simulink model "fwv_fulatti"  (R2021b)
settings: Solver=ode15s  StartTime=0.0  StopTime=10  FixedStep=0.01  MaxStep=0.01  RelTol=1e-3  AbsTol=1e-3  EnableMultiTasking=on
model workspace (MATLAB code in the model file):
  | p0=[0 0 0];
values from neighbouring files (symbols this model uses):
  A_D = 1.5    [main.m]    (also in param.m; params.m)
  A_L = 1.8    [main.m]    (also in param.m; params.m)
  c_bar = S/R    (= 0.0357142857143)    [main.m]    (also in param.m = 0.0251327412287; params.m)
  C_D0 = 0.45    [main.m]    (also in param.m; params.m)
  m = 2    [rbf_pid.m]
  r00 = double(int(f,[0,1]))    [main.m]    (also in param.m = 1; params.m = 0.933333333333)
  r11 = double(int(x*f,[0,1]))    [main.m]    (also in param.m = double(int(curv(x)*(x+1/9),0,1)); params.m = 0.481185185185)
  r22 = double(int(x^2*f,[0,1]))    [main.m]    (also in param.m = double(int(curv(x)*(x+1/9)^2,0,1)); params.m = 0.304750617284)
  r33 = double(int(x^3*f,[0,1]))    [main.m]    (also in param.m = double(int(curv(x)*(x+1/9)^3,0,1)); params.m = 0.218568691358)
  r_cp = Rw*r33/r22    [main.m]    (also in param.m; params.m = 0.10758076225)
  rho = 1.205    [main.m]    (also in param.m; params.m)
  Rw = 0.15    [main.m]    (also in param.m = 0.075; params.m)
  z00 = double(int(f^2,[0,1]))    [main.m]    (also in param.m = double(int(curv(x)^2,0,1)); params.m = 1.00177777778)
  z11 = double(int(x*f^2,[0,1]))    [main.m]    (also in param.m = double(int(curv(x)^2*(x+1/9),0,1)); params.m = 0.484918518519)
  z22 = double(int(x^2*f^2,[0,1]))    [main.m]    (also in param.m = double(int(curv(x)^2*(x+1/9)^2,0,1)); params.m = 0.28785382716)
  zrd = double(int(f^4,[0,1]))    [main.m]    (also in param.m = double(int(curv(x)^4,0,1)); params.m = 1.29333866667)
undefined symbols (not defined in the file or in its folder): X, Y, Z
libraries: sm_lib x57, nesl_utility x45, vrlib x3, slpidlib x2
(part 3 of 3)

== system fwv_fulatti/Controller/Outer PD ==
  ep : Inport
  ev : Inport  Port=2
  a : Inport  Port=3
  Demux : Demux  Outputs=3
  Demux1 : Demux  Outputs=3
  Demux2 : Demux  Outputs=3
  x PD : Subsystem  mask{Kp=6, Ki=0, Kd=3}
  x PID : slpidlib/PID Controller  Commented=on  Controller=PID  Form=Parallel  TimeDomain=Continuous-time  UseExternalTs=off  SampleTime=-1  IntegratorMethod=Forward Euler  FilterMethod=Forward Euler  ControllerParametersSource=internal  P=0.5  I=0  D=0.1  UseFilter=on  N=25  TunerSelectOption=Transfer Function Based (PID Tuner App)  InitialConditionSource=internal  InitialConditionForIntegrator=0  InitialConditionForFilter=0  DifferentiatorICPrevScaledInput=0  ExternalReset=none  TrackingMode=off  Kt=1  LimitOutput=off  SatLimitsSource=internal  UpperSaturationLimit=0.5  LowerSaturationLimit=-0.5  LinearizeAsGain=on  AntiWindupMode=none  Kb=1  POutMin=[]  POutMax=[]  IOutMin=[]  IOutMax=[]  DOutMin=[]  DOutMax=[]  NOutMin=[]  NOutMax=[]  SumOutDataTypeStr=double  SumOutMin=[]  SumOutMax=[]  SaturationOutMin=[]  SaturationOutMax=[]  PParamMin=[]  PParamMax=[]  IParamMin=[]  IParamMax=[]  DParamMin=[]  DParamMax=[]  NParamMin=[]  NParamMax=[]  KbParamMin=[]  KbParamMax=[]  KtParamMin=[]  KtParamMax=[]  KbOutMin=[]  KbOutMax=[]  KtOutMin=[]  KtOutMax=[]  IntegratorOutMin=[]  IntegratorOutMax=[]  FilterOutMin=[]  FilterOutMax=[]  SumI1OutMin=[]  SumI1OutMax=[]  SumI2OutMin=[]  SumI2OutMax=[]  SumI3OutMin=[]  SumI3OutMax=[]  SumI4OutMin=[]  SumI4OutMax=[]  SumDOutMin=[]  SumDOutMax=[]  DifferentiatorOutMin=[]  DifferentiatorOutMax=[]  FilterDiffOutCoefMin=[]  FilterDiffOutCoefMax=[]  ReciprocalOutMin=[]  ReciprocalOutMax=[]  SumDenOutMin=[]  SumDenOutMax=[]  SumNumOutMin=[]  SumNumOutMax=[]  DivideOutMin=[]  DivideOutMax=[]  UdiffTsProdOutMin=[]  UdiffTsProdOutMax=[]  NTsProdOutMin=[]  NTsProdOutMax=[]  UintegralTsProdOutMin=[]  UintegralTsProdOutMax=[]  UngainTsProdOutMin=[]  UngainTsProdOutMax=[]  IntegratorContinuousStateAttributes=''  IntegratorStateMustResolveToSignalObject=off  IntegratorRTWStateStorageClass=Auto  FilterContinuousStateAttributes=''  FilterStateMustResolveToSignalObject=off  FilterRTWStateStorageClass=Auto  ParallelPVariant=InternalParameters  IdealPVariant=Disabled  IVariant=InternalParameters  DVariant=InternalParameters  IntegratorVariant=Continuous  SatVariant=Disabled  AWVariant=Passthrough  PCopyVariant=Disabled  TRVariant=Disabled  FdbkBlocksVariant=Forward  IdealPFdbkVariant=Disabled  SatFdbkVariant=Disabled  DerivativeFilterVariant=ContFilter  NVariant=InternalParameters  NCopyVariant=Disabled  FilterICVariant=InternalICsFilter  IntegratorICVariant=InternalICs  ExternalResetVariant=Disabled  TRSumVariant=Passthrough  SumFdbkVariant=Disabled  SumVariant=Sum_PID  TsampFilterVariant=InternalTs  TsampNgainVariant=Passthrough  TsampIntegralVariant=Passthrough  ExternalSaturationOutDataTypeStr=Inherit: Same as second input
  y PD : Subsystem  mask{Kp=6, Ki=0, Kd=6}
  y PID : slpidlib/PID Controller  Commented=on  Controller=PID  Form=Parallel  TimeDomain=Continuous-time  UseExternalTs=off  SampleTime=-1  IntegratorMethod=Forward Euler  FilterMethod=Forward Euler  ControllerParametersSource=internal  P=0.3  I=0  D=0.3  UseFilter=on  N=25  TunerSelectOption=Transfer Function Based (PID Tuner App)  InitialConditionSource=internal  InitialConditionForIntegrator=0  InitialConditionForFilter=0  DifferentiatorICPrevScaledInput=0  ExternalReset=none  TrackingMode=off  Kt=1  LimitOutput=off  SatLimitsSource=internal  UpperSaturationLimit=0.5  LowerSaturationLimit=-0.5  LinearizeAsGain=on  AntiWindupMode=none  Kb=1  POutMin=[]  POutMax=[]  IOutMin=[]  IOutMax=[]  DOutMin=[]  DOutMax=[]  NOutMin=[]  NOutMax=[]  SumOutMin=[]  SumOutMax=[]  SaturationOutMin=[]  SaturationOutMax=[]  PParamMin=[]  PParamMax=[]  IParamMin=[]  IParamMax=[]  DParamMin=[]  DParamMax=[]  NParamMin=[]  NParamMax=[]  KbParamMin=[]  KbParamMax=[]  KtParamMin=[]  KtParamMax=[]  KbOutMin=[]  KbOutMax=[]  KtOutMin=[]  KtOutMax=[]  IntegratorOutMin=[]  IntegratorOutMax=[]  FilterOutMin=[]  FilterOutMax=[]  SumI1OutMin=[]  SumI1OutMax=[]  SumI2OutMin=[]  SumI2OutMax=[]  SumI3OutMin=[]  SumI3OutMax=[]  SumI4OutMin=[]  SumI4OutMax=[]  SumDOutMin=[]  SumDOutMax=[]  DifferentiatorOutMin=[]  DifferentiatorOutMax=[]  FilterDiffOutCoefMin=[]  FilterDiffOutCoefMax=[]  ReciprocalOutMin=[]  ReciprocalOutMax=[]  SumDenOutMin=[]  SumDenOutMax=[]  SumNumOutMin=[]  SumNumOutMax=[]  DivideOutMin=[]  DivideOutMax=[]  UdiffTsProdOutMin=[]  UdiffTsProdOutMax=[]  NTsProdOutMin=[]  NTsProdOutMax=[]  UintegralTsProdOutMin=[]  UintegralTsProdOutMax=[]  UngainTsProdOutMin=[]  UngainTsProdOutMax=[]  IntegratorContinuousStateAttributes=''  IntegratorStateMustResolveToSignalObject=off  IntegratorRTWStateStorageClass=Auto  FilterContinuousStateAttributes=''  FilterStateMustResolveToSignalObject=off  FilterRTWStateStorageClass=Auto  ParallelPVariant=InternalParameters  IdealPVariant=Disabled  IVariant=InternalParameters  DVariant=InternalParameters  IntegratorVariant=Continuous  SatVariant=Disabled  AWVariant=Passthrough  PCopyVariant=Disabled  TRVariant=Disabled  FdbkBlocksVariant=Forward  IdealPFdbkVariant=Disabled  SatFdbkVariant=Disabled  DerivativeFilterVariant=ContFilter  NVariant=InternalParameters  NCopyVariant=Disabled  FilterICVariant=InternalICsFilter  IntegratorICVariant=InternalICs  ExternalResetVariant=Disabled  TRSumVariant=Passthrough  SumFdbkVariant=Disabled  SumVariant=Sum_PID  TsampFilterVariant=InternalTs  TsampNgainVariant=Passthrough  TsampIntegralVariant=Passthrough  ExternalSaturationOutDataTypeStr=Inherit: Same as second input
  z PD : Subsystem  mask{Kp=10, Ki=0, Kd=4}
  mux : Outport
  muy : Outport  Port=2
  muz : Outport  Port=3
  wires:
  ep/1 -> Demux/1
  ev/1 -> Demux1/1
  x PD/1(Out1) -> mux/1
  y PD/1(Out1) -> muy/1
  z PD/1(Out1) -> muz/1
  a/1 -> Demux2/1
  Demux1/2 -> y PD/2(In2)
  Demux2/3 -> z PD/3(In3)
  Demux2/2 -> y PD/3(In3)
  Demux1/1 -> x PD/2(In2)
  Demux1/3 -> z PD/2(In2)
  Demux/3 -> z PD/1(In1)
  Demux2/1 -> x PD/3(In3)
  Demux/1 -> x PD/1(In1)
  Demux/2 -> y PD/1(In1)

== system fwv_fulatti/Controller/R to euler ==
  R : Inport
  Mux : Mux  Inputs=3
  R to X-Y-Z Extrinsic : Subsystem  mask(Rotation Matrix to X-Y-Z Extrinsic){}
      mask help: Computes roll / pitch / yaw values assuming they correspond to X, Y, and Z rotations, applied in that order and using extrinsic rotations (rotations applied about the fixed axes of the base frame). Does not handle case where Y (pitch) rotation is +/-90 degrees.
  Terminator : Terminator
  rad2deg : Gain  Gain=180/pi
  wires:
  R/1 -> R to X-Y-Z Extrinsic/1(R)
  R to X-Y-Z Extrinsic/2(pitch) -> Mux/2
  Mux/1 -> rad2deg/1
  rad2deg/1 -> Terminator/1
  R to X-Y-Z Extrinsic/1(roll) -> Mux/1
  R to X-Y-Z Extrinsic/3(yaw) -> Mux/3

== system fwv_fulatti/Controller/Rd to euler ==
  R : Inport
  Mux : Mux  Inputs=3
  R to X-Y-Z Extrinsic : Subsystem  mask(Rotation Matrix to X-Y-Z Extrinsic){}
      mask help: Computes roll / pitch / yaw values assuming they correspond to X, Y, and Z rotations, applied in that order and using extrinsic rotations (rotations applied about the fixed axes of the base frame). Does not handle case where Y (pitch) rotation is +/-90 degrees.
  Terminator : Terminator
  rad2deg : Gain  Gain=180/pi
  wires:
  rad2deg/1 -> Terminator/1
  R/1 -> R to X-Y-Z Extrinsic/1(R)
  Mux/1 -> rad2deg/1
  R to X-Y-Z Extrinsic/3(yaw) -> Mux/3
  R to X-Y-Z Extrinsic/1(roll) -> Mux/1
  R to X-Y-Z Extrinsic/2(pitch) -> Mux/2

== system fwv_fulatti/Controller/adaptive mapping estimator ==
  mu : Inport
  Integrator : Integrator  InitialCondition=0.05
  update k_hat : MATLAB Function  TreatAsAtomicUnit=on
  k_hat : Outport
  wires:
  update k_hat/1(k_hat_dot) -> Integrator/1
  mu/1 -> update k_hat/1(mu)
  Integrator/1 -> update k_hat/2(k_hat), k_hat/1

== system fwv_fulatti/Controller/averaged R to euler ==
  R : Inport
  Mux : Mux  Inputs=3
  R to X-Y-Z Extrinsic : Subsystem  mask(Rotation Matrix to X-Y-Z Extrinsic){}
      mask help: Computes roll / pitch / yaw values assuming they correspond to X, Y, and Z rotations, applied in that order and using extrinsic rotations (rotations applied about the fixed axes of the base frame). Does not handle case where Y (pitch) rotation is +/-90 degrees.
  Terminator : Terminator
  rad2deg : Gain  Gain=180/pi
  wires:
  R/1 -> R to X-Y-Z Extrinsic/1(R)
  R to X-Y-Z Extrinsic/2(pitch) -> Mux/2
  Mux/1 -> rad2deg/1
  rad2deg/1 -> Terminator/1
  R to X-Y-Z Extrinsic/1(roll) -> Mux/1
  R to X-Y-Z Extrinsic/3(yaw) -> Mux/3

== system fwv_fulatti/Controller/period averaging ==
  in : Inport
  MATLAB Function : MATLAB Function  TreatAsAtomicUnit=on
  Mean : Subsystem
  Mean1 : Outport
  wires:
  in/1 -> Mean/1(In1)
  Mean/1(Out1) -> MATLAB Function/1(R_raw)
  MATLAB Function/1(R_mean) -> Mean1/1

== system fwv_fulatti/Body/LEFT WING/Subsystem1 ==
  Gain : Gain  Gain=-1
  LWing-root in world : sm_lib/Frames and Transforms/Transform Sensor  MeasurementFrame=NonRotatingFollower  SenseAngle=off  SenseAxis=off  SenseAngle1=off  SenseAngle2=off  SenseAngle3=off  SenseQ=off  SenseR=off  SenseOmegaX=on  SenseOmegaY=on  SenseOmegaZ=off  SenseOmega1=off  SenseOmega2=off  SenseOmega3=off  SenseQDot=off  SenseRDot=off  SenseAlphaX=off  SenseAlphaY=off  SenseAlphaZ=off  SenseAlpha1=off  SenseAlpha2=off  SenseAlpha3=off  SenseQDDot=off  SenseRDDot=off  SenseX=off  SenseY=off  SenseZ=off  SenseRad=off  SenseAzim=off  SenseDist=off  SenseInc=off  SenseXDot=on  SenseYDot=on  SenseZDot=off  SenseRadDot=off  SenseAzimDot=off  SenseDistDot=off  SenseIncDot=off  SenseXDDot=off  SenseYDDot=off  SenseZDDot=off  SenseRadDDot=off  SenseAzimDDot=off  SenseDistDDot=off  SenseIncDDot=off
  Mux : Mux
  PS-Simulink Converter{,1..3} (4 alike) : nesl_utility/PS-Simulink Converter  PhysicalDomain=network_engine_domain  SubClassName=ps_output  LeftPortType=input  RightPortType=output  PseudoPeriodic=off  Frequencies=[]  Unit=inherit  AffineConversion=off
      settings: SourceProductBaseCode=PW,SS
  W : PMIOPort  Side=Left
  WT : PMIOPort  Port=2  Side=Left
  le0 : Outport
  wires:
  Mux/1 -> le0/1
  Gain/1 -> Mux/2
  PS-Simulink Converter1/1 -> Mux/3
  PS-Simulink Converter3/1 -> Gain/1
  PS-Simulink Converter2/1 -> Mux/1
  PS-Simulink Converter/1 -> Mux/4
  connections:
  W/RConn1 -- LWing-root in world/LConn1
  WT/RConn1 -- LWing-root in world/RConn1
  LWing-root in world/RConn2 -- PS-Simulink Converter/LConn1
  LWing-root in world/RConn3 -- PS-Simulink Converter1/LConn1
  LWing-root in world/RConn4 -- PS-Simulink Converter2/LConn1
  LWing-root in world/RConn5 -- PS-Simulink Converter3/LConn1

== system fwv_fulatti/Body/RIGHT WING/Subsystem1 ==
  Gain : Gain  Gain=-1
  LWing-root in world : sm_lib/Frames and Transforms/Transform Sensor  MeasurementFrame=NonRotatingFollower  SenseAngle=off  SenseAxis=off  SenseAngle1=off  SenseAngle2=off  SenseAngle3=off  SenseQ=off  SenseR=off  SenseOmegaX=on  SenseOmegaY=on  SenseOmegaZ=off  SenseOmega1=off  SenseOmega2=off  SenseOmega3=off  SenseQDot=off  SenseRDot=off  SenseAlphaX=off  SenseAlphaY=off  SenseAlphaZ=off  SenseAlpha1=off  SenseAlpha2=off  SenseAlpha3=off  SenseQDDot=off  SenseRDDot=off  SenseX=off  SenseY=off  SenseZ=off  SenseRad=off  SenseAzim=off  SenseDist=off  SenseInc=off  SenseXDot=on  SenseYDot=on  SenseZDot=off  SenseRadDot=off  SenseAzimDot=off  SenseDistDot=off  SenseIncDot=off  SenseXDDot=off  SenseYDDot=off  SenseZDDot=off  SenseRadDDot=off  SenseAzimDDot=off  SenseDistDDot=off  SenseIncDDot=off
  Mux : Mux
  PS-Simulink Converter{,1..3} (4 alike) : nesl_utility/PS-Simulink Converter  PhysicalDomain=network_engine_domain  SubClassName=ps_output  LeftPortType=input  RightPortType=output  PseudoPeriodic=off  Frequencies=[]  Unit=inherit  AffineConversion=off
      settings: SourceProductBaseCode=PW,SS
  W : PMIOPort  Side=Left
  WT : PMIOPort  Port=2  Side=Left
  le0 : Outport
  wires:
  Mux/1 -> le0/1
  Gain/1 -> Mux/2
  PS-Simulink Converter1/1 -> Mux/3
  PS-Simulink Converter3/1 -> Gain/1
  PS-Simulink Converter2/1 -> Mux/1
  PS-Simulink Converter/1 -> Mux/4
  connections:
  W/RConn1 -- LWing-root in world/LConn1
  WT/RConn1 -- LWing-root in world/RConn1
  LWing-root in world/RConn2 -- PS-Simulink Converter/LConn1
  LWing-root in world/RConn3 -- PS-Simulink Converter1/LConn1
  LWing-root in world/RConn4 -- PS-Simulink Converter2/LConn1
  LWing-root in world/RConn5 -- PS-Simulink Converter3/LConn1

== system fwv_fulatti/Controller/Inner PD/get P ==
  eR : Inport
  Add : Sum  Inputs=+++
  Cross Product : vrlib/Utilities/Cross Product
  Cross Product1 : vrlib/Utilities/Cross Product
  Cross Product2 : vrlib/Utilities/Cross Product
  One : Constant  Value=[1;0;0]  OutDataTypeStr=Inherit: Inherit via back propagation
  One1 : Constant  Value=[0;1;0]  OutDataTypeStr=Inherit: Inherit via back propagation
  One2 : Constant  Value=[0;0;1]  OutDataTypeStr=Inherit: Inherit via back propagation
  Product : Product  Multiplication=Matrix(*)
  Product1 : Product  Multiplication=Matrix(*)
  Product2 : Product  Multiplication=Matrix(*)
  Out : Outport
  wires:
  One/1 -> Product/2, Cross Product/1
  One1/1 -> Cross Product1/1, Product1/2
  One2/1 -> Cross Product2/1, Product2/2
  eR/1 -> Product/1, Product1/1, Product2/1
  Cross Product/1 -> Add/1
  Cross Product1/1 -> Add/2
  Cross Product2/1 -> Add/3
  Add/1 -> Out/1
  Product/1 -> Cross Product/2
  Product1/1 -> Cross Product1/2
  Product2/1 -> Cross Product2/2

== system fwv_fulatti/Controller/Inner PD/to euler1 ==
  R : Inport
  Mux : Mux  Inputs=3
  R to X-Y-Z Extrinsic : Subsystem  mask(Rotation Matrix to X-Y-Z Extrinsic){}
      mask help: Computes roll / pitch / yaw values assuming they correspond to X, Y, and Z rotations, applied in that order and using extrinsic rotations (rotations applied about the fixed axes of the base frame). Does not handle case where Y (pitch) rotation is +/-90 degrees.
  Terminator : Terminator
  rad2deg : Gain  Gain=180/pi
  wires:
  rad2deg/1 -> Terminator/1
  R/1 -> R to X-Y-Z Extrinsic/1(R)
  Mux/1 -> rad2deg/1
  R to X-Y-Z Extrinsic/3(yaw) -> Mux/3
  R to X-Y-Z Extrinsic/1(roll) -> Mux/1
  R to X-Y-Z Extrinsic/2(pitch) -> Mux/2

== system fwv_fulatti/Controller/Outer PD/x PD ==
  In1 : Inport
  In2 : Inport  Port=2
  In3 : Inport  Port=3
  Add : Sum  Inputs=++++
  Constant : Constant  Value=Kp
  Constant1 : Constant  Value=Ki
  Constant2 : Constant  Value=Kd
  Gain : Gain
  Integrator Limited : Integrator  UpperSaturationLimit=1  LowerSaturationLimit=0
  Product : Product
  Product1 : Product
  Product2 : Product
  Scope : Scope  NumInputPorts=2
  Out1 : Outport
  wires:
  Add/1 -> Out1/1
  In1/1 -> Product1/2, Product/2
  Product/1 -> Scope/1, Add/1
  Constant/1 -> Product/1
  Product2/1 -> Scope/2, Add/3
  In2/1 -> Product2/2
  Constant2/1 -> Product2/1
  Integrator Limited/1 -> Add/2
  Product1/1 -> Integrator Limited/1
  Constant1/1 -> Product1/1
  In3/1 -> Gain/1
  Gain/1 -> Add/4

== system fwv_fulatti/Controller/Outer PD/y PD ==
  In1 : Inport
  In2 : Inport  Port=2
  In3 : Inport  Port=3
  Add : Sum  Inputs=++++
  Constant : Constant  Value=Kp
  Constant1 : Constant  Value=Ki
  Constant2 : Constant  Value=Kd
  Gain : Gain
  Integrator Limited : Integrator  UpperSaturationLimit=1  LowerSaturationLimit=0
  Product : Product
  Product1 : Product
  Product2 : Product
  Out1 : Outport
  wires:
  Add/1 -> Out1/1
  In1/1 -> Product1/2, Product/2
  Product/1 -> Add/1
  Constant/1 -> Product/1
  Product2/1 -> Add/3
  In2/1 -> Product2/2
  Constant2/1 -> Product2/1
  Integrator Limited/1 -> Add/2
  Product1/1 -> Integrator Limited/1
  Constant1/1 -> Product1/1
  In3/1 -> Gain/1
  Gain/1 -> Add/4

== system fwv_fulatti/Controller/Outer PD/z PD ==
  In1 : Inport
  In2 : Inport  Port=2
  In3 : Inport  Port=3
  Add : Sum  Inputs=++++
  Constant : Constant  Value=Kp
  Constant1 : Constant  Value=Ki
  Constant2 : Constant  Value=Kd
  Integrator Limited : Integrator  UpperSaturationLimit=5  LowerSaturationLimit=-5
  Product : Product
  Product1 : Product
  Product2 : Product
  Scope : Scope
  Scope1 : Scope
  Out1 : Outport
  wires:
  Add/1 -> Out1/1
  In1/1 -> Product1/2, Scope/1, Product/2
  Product/1 -> Add/1
  Constant/1 -> Product/1
  Product2/1 -> Add/3
  In2/1 -> Scope1/1, Product2/2
  Constant2/1 -> Product2/1
  Integrator Limited/1 -> Add/2
  Product1/1 -> Integrator Limited/1
  Constant1/1 -> Product1/1
  In3/1 -> Add/4

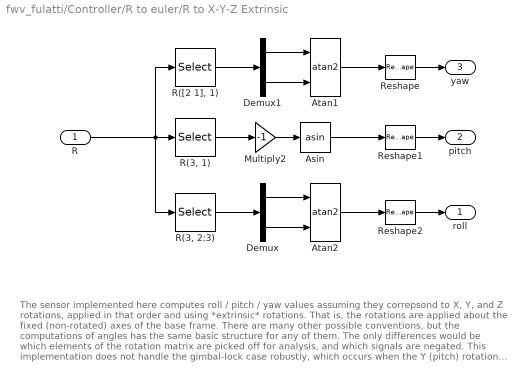
== system fwv_fulatti/Controller/R to euler/R to X-Y-Z Extrinsic ==
  note: The sensor implemented here computes roll / pitch / yaw values assuming they correpsond to X, Y, and Z rotations, applied in that order and using  *extrinsic* rotations.  That is, the rotations are applied about the fixed (non-rotated) axes of the base frame.   There are many other possible conventions, but the computations of angles has the same basic structure for any of them.  The only differences would be which elements of the rotation matrix are picked off for analysis, and which signals are negated.
      |
      | This implementation does not handle the gimbal-lock case robustly, which occurs when the Y (pitch) rotation is +/-90 degrees.  Handling this case requires a more complex computation,
      | but it can be done with a few more trig blocks and selectors.
  R : Inport
  Asin : Trigonometry  Operator=asin
  Atan1 : Trigonometry  Operator=atan2
  Atan2 : Trigonometry  Operator=atan2
  Demux : Demux  Outputs=2
  Demux1 : Demux  Outputs=2
  Multiply2 : Gain  Gain=-1
  "R(3, 1)" : Selector  NumberOfDimensions=2  InputPortWidth=3  IndexOptions=Index vector (dialog),Index vector (dialog)  Indices=3,1  OutputSizes=1,1
  "R(3, 2:3)" : Selector  NumberOfDimensions=2  InputPortWidth=3  IndexOptions=Index vector (dialog),Index vector (dialog)  Indices=3,[2 3]  OutputSizes=1,1
  "R([2 1], 1)" : Selector  NumberOfDimensions=2  InputPortWidth=3  IndexOptions=Index vector (dialog),Index vector (dialog)  Indices=[2 1],1  OutputSizes=1,1
  Reshape : Reshape
  Reshape1 : Reshape
  Reshape2 : Reshape  OutputDimensionality=Customize  OutputDimensions=1
  roll : Outport  VectorParamsAs1DForOutWhenUnconnected=off
  pitch : Outport  Port=2  VectorParamsAs1DForOutWhenUnconnected=off
  yaw : Outport  Port=3  VectorParamsAs1DForOutWhenUnconnected=off
  wires:
  Demux/1 -> Atan2/1
  Demux1/2 -> Atan1/2
  Demux/2 -> Atan2/2
  Atan2/1 -> Reshape2/1
  "R(3, 1)"/1 -> Multiply2/1
  Asin/1 -> Reshape1/1
  R/1 -> "R(3, 1)"/1, "R(3, 2:3)"/1, "R([2 1], 1)"/1
  Demux1/1 -> Atan1/1
  "R([2 1], 1)"/1 -> Demux1/1
  Multiply2/1 -> Asin/1
  "R(3, 2:3)"/1 -> Demux/1
  Atan1/1 -> Reshape/1
  Reshape/1 -> yaw/1
  Reshape1/1 -> pitch/1
  Reshape2/1 -> roll/1

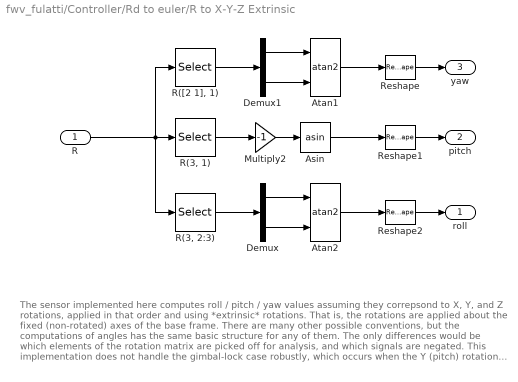
== system fwv_fulatti/Controller/Rd to euler/R to X-Y-Z Extrinsic ==
  note: The sensor implemented here computes roll / pitch / yaw values assuming they correpsond to X, Y, and Z rotations, applied in that order and using  *extrinsic* rotations.  That is, the rotations are applied about the fixed (non-rotated) axes of the base frame.   There are many other possible conventions, but the computations of angles has the same basic structure for any of them.  The only differences would be which elements of the rotation matrix are picked off for analysis, and which signals are negated.
      |
      | This implementation does not handle the gimbal-lock case robustly, which occurs when the Y (pitch) rotation is +/-90 degrees.  Handling this case requires a more complex computation,
      | but it can be done with a few more trig blocks and selectors.
  R : Inport
  Asin : Trigonometry  Operator=asin
  Atan1 : Trigonometry  Operator=atan2
  Atan2 : Trigonometry  Operator=atan2
  Demux : Demux  Outputs=2
  Demux1 : Demux  Outputs=2
  Multiply2 : Gain  Gain=-1
  "R(3, 1)" : Selector  NumberOfDimensions=2  InputPortWidth=3  IndexOptions=Index vector (dialog),Index vector (dialog)  Indices=3,1  OutputSizes=1,1
  "R(3, 2:3)" : Selector  NumberOfDimensions=2  InputPortWidth=3  IndexOptions=Index vector (dialog),Index vector (dialog)  Indices=3,[2 3]  OutputSizes=1,1
  "R([2 1], 1)" : Selector  NumberOfDimensions=2  InputPortWidth=3  IndexOptions=Index vector (dialog),Index vector (dialog)  Indices=[2 1],1  OutputSizes=1,1
  Reshape : Reshape
  Reshape1 : Reshape
  Reshape2 : Reshape  OutputDimensionality=Customize  OutputDimensions=1
  roll : Outport  VectorParamsAs1DForOutWhenUnconnected=off
  pitch : Outport  Port=2  VectorParamsAs1DForOutWhenUnconnected=off
  yaw : Outport  Port=3  VectorParamsAs1DForOutWhenUnconnected=off
  wires:
  Demux/1 -> Atan2/1
  Demux1/2 -> Atan1/2
  Demux/2 -> Atan2/2
  Atan2/1 -> Reshape2/1
  "R(3, 1)"/1 -> Multiply2/1
  Asin/1 -> Reshape1/1
  R/1 -> "R(3, 1)"/1, "R(3, 2:3)"/1, "R([2 1], 1)"/1
  Demux1/1 -> Atan1/1
  "R([2 1], 1)"/1 -> Demux1/1
  Multiply2/1 -> Asin/1
  "R(3, 2:3)"/1 -> Demux/1
  Atan1/1 -> Reshape/1
  Reshape/1 -> yaw/1
  Reshape1/1 -> pitch/1
  Reshape2/1 -> roll/1

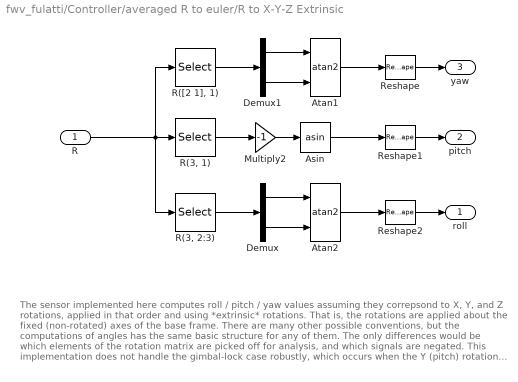
== system fwv_fulatti/Controller/averaged R to euler/R to X-Y-Z Extrinsic ==
  note: The sensor implemented here computes roll / pitch / yaw values assuming they correpsond to X, Y, and Z rotations, applied in that order and using  *extrinsic* rotations.  That is, the rotations are applied about the fixed (non-rotated) axes of the base frame.   There are many other possible conventions, but the computations of angles has the same basic structure for any of them.  The only differences would be which elements of the rotation matrix are picked off for analysis, and which signals are negated.
      |
      | This implementation does not handle the gimbal-lock case robustly, which occurs when the Y (pitch) rotation is +/-90 degrees.  Handling this case requires a more complex computation,
      | but it can be done with a few more trig blocks and selectors.
  R : Inport
  Asin : Trigonometry  Operator=asin
  Atan1 : Trigonometry  Operator=atan2
  Atan2 : Trigonometry  Operator=atan2
  Demux : Demux  Outputs=2
  Demux1 : Demux  Outputs=2
  Multiply2 : Gain  Gain=-1
  "R(3, 1)" : Selector  NumberOfDimensions=2  InputPortWidth=3  IndexOptions=Index vector (dialog),Index vector (dialog)  Indices=3,1  OutputSizes=1,1
  "R(3, 2:3)" : Selector  NumberOfDimensions=2  InputPortWidth=3  IndexOptions=Index vector (dialog),Index vector (dialog)  Indices=3,[2 3]  OutputSizes=1,1
  "R([2 1], 1)" : Selector  NumberOfDimensions=2  InputPortWidth=3  IndexOptions=Index vector (dialog),Index vector (dialog)  Indices=[2 1],1  OutputSizes=1,1
  Reshape : Reshape
  Reshape1 : Reshape
  Reshape2 : Reshape  OutputDimensionality=Customize  OutputDimensions=1
  roll : Outport  VectorParamsAs1DForOutWhenUnconnected=off
  pitch : Outport  Port=2  VectorParamsAs1DForOutWhenUnconnected=off
  yaw : Outport  Port=3  VectorParamsAs1DForOutWhenUnconnected=off
  wires:
  Demux/1 -> Atan2/1
  Demux1/2 -> Atan1/2
  Demux/2 -> Atan2/2
  Atan2/1 -> Reshape2/1
  "R(3, 1)"/1 -> Multiply2/1
  Asin/1 -> Reshape1/1
  R/1 -> "R(3, 1)"/1, "R(3, 2:3)"/1, "R([2 1], 1)"/1
  Demux1/1 -> Atan1/1
  "R([2 1], 1)"/1 -> Demux1/1
  Multiply2/1 -> Asin/1
  "R(3, 2:3)"/1 -> Demux/1
  Atan1/1 -> Reshape/1
  Reshape/1 -> yaw/1
  Reshape1/1 -> pitch/1
  Reshape2/1 -> roll/1

== system fwv_fulatti/Controller/period averaging/Mean ==
  In1 : Inport
  Add : Sum  Inputs=+-
  Gain : Gain  Gain=1/0.04
  Integrator : Integrator  ZeroCross=off
  Transport Delay : TransportDelay  DelayTime=0.04  InitialOutput=[0,0,0;0,0,0;0,0,0]
  Out1 : Outport
  wires:
  In1/1 -> Integrator/1
  Integrator/1 -> Transport Delay/1, Add/1
  Add/1 -> Gain/1
  Gain/1 -> Out1/1
  Transport Delay/1 -> Add/2

== system fwv_fulatti/Controller/Inner PD/to euler1/R to X-Y-Z Extrinsic ==
  note: The sensor implemented here computes roll / pitch / yaw values assuming they correpsond to X, Y, and Z rotations, applied in that order and using  *extrinsic* rotations.  That is, the rotations are applied about the fixed (non-rotated) axes of the base frame.   There are many other possible conventions, but the computations of angles has the same basic structure for any of them.  The only differences would be which elements of the rotation matrix are picked off for analysis, and which signals are negated.
      |
      | This implementation does not handle the gimbal-lock case robustly, which occurs when the Y (pitch) rotation is +/-90 degrees.  Handling this case requires a more complex computation,
      | but it can be done with a few more trig blocks and selectors.
  R : Inport
  Asin : Trigonometry  Operator=asin
  Atan1 : Trigonometry  Operator=atan2
  Atan2 : Trigonometry  Operator=atan2
  Demux : Demux  Outputs=2
  Demux1 : Demux  Outputs=2
  Multiply2 : Gain  Gain=-1
  "R(3, 1)" : Selector  NumberOfDimensions=2  InputPortWidth=3  IndexOptions=Index vector (dialog),Index vector (dialog)  Indices=3,1  OutputSizes=1,1
  "R(3, 2:3)" : Selector  NumberOfDimensions=2  InputPortWidth=3  IndexOptions=Index vector (dialog),Index vector (dialog)  Indices=3,[2 3]  OutputSizes=1,1
  "R([2 1], 1)" : Selector  NumberOfDimensions=2  InputPortWidth=3  IndexOptions=Index vector (dialog),Index vector (dialog)  Indices=[2 1],1  OutputSizes=1,1
  Reshape : Reshape
  Reshape1 : Reshape
  Reshape2 : Reshape  OutputDimensionality=Customize  OutputDimensions=1
  roll : Outport  VectorParamsAs1DForOutWhenUnconnected=off
  pitch : Outport  Port=2  VectorParamsAs1DForOutWhenUnconnected=off
  yaw : Outport  Port=3  VectorParamsAs1DForOutWhenUnconnected=off
  wires:
  Demux/1 -> Atan2/1
  Demux1/2 -> Atan1/2
  Demux/2 -> Atan2/2
  Atan2/1 -> Reshape2/1
  "R(3, 1)"/1 -> Multiply2/1
  Asin/1 -> Reshape1/1
  R/1 -> "R(3, 1)"/1, "R(3, 2:3)"/1, "R([2 1], 1)"/1
  Demux1/1 -> Atan1/1
  "R([2 1], 1)"/1 -> Demux1/1
  Multiply2/1 -> Asin/1
  "R(3, 2:3)"/1 -> Demux/1
  Atan1/1 -> Reshape/1
  Reshape/1 -> yaw/1
  Reshape1/1 -> pitch/1
  Reshape2/1 -> roll/1

== matlab function fwv_fulatti/Body/LEFT WING/left aero force and moment ==
  data: le0 input; F_N output; alpha input; M_rd output; M_ae output; d_cp output; rot_dot input; A_L parameter; A_D parameter; C_D0 parameter; rho parameter; c_bar parameter; Rw parameter; r22 parameter; r11 parameter; r00 parameter; z22 parameter; z11 parameter; z00 parameter; zrd parameter
function [F_N, M_rd, M_ae, d_cp] = fcn(le0, alpha, rot_dot, A_L, A_D, C_D0, rho, c_bar, Rw, r22, r11, r00, z22, z11, z00, zrd)
a2=le0(3)^2+le0(4)^2;
a1=2*(le0(1)*le0(3)+le0(2)*le0(4));
a0=le0(1)^2+le0(2)^2;
C_L=A_L*sin(2*alpha);
C_D=C_D0+A_D*(1-cos(2*alpha));
C_N=C_L*cos(alpha)+C_D*sin(alpha);
C_A=C_L*sin(alpha)-C_D*cos(alpha);
F_N = -0.5*rho*C_N*c_bar*(a2*Rw^3*r22+a1*Rw^2*r11+a0*Rw*r00);
d_cp_=0.82/pi*(mod(abs(alpha),pi))+0.05;
M_ae=0.5*rho*C_N*c_bar^2*d_cp_*(a2*Rw^3*z22+a1*Rw^2*z11+a0*Rw*z00);
if F_N==0
    d_cp=-0.51*c_bar;
else
    d_cp = M_ae/F_N;
end
M_rd=-0.125*rho*5*rot_dot*abs(rot_dot)*Rw*c_bar^4*zrd;

== matlab function fwv_fulatti/Body/RIGHT WING/AoA1 ==
  data: le0 input; alpha output; rot input; Rw parameter; r33 parameter; r22 parameter
function alpha = fcn(le0, rot, Rw, r33, r22)
rcp = -Rw*r33/r22;
vi = le0(1)+le0(3)*rcp;
vo = le0(2)+le0(4)*rcp;
if vi~=0
    alpha = -rot + sign(vi)*pi/2 - atan(vo/vi);
else
    alpha = 0;
end

== matlab function fwv_fulatti/Body/RIGHT WING/right aero force and moment ==
  data: le0 input; F_N output; alpha input; M_rd output; d_cp output; rot_dot input; A_L parameter; A_D parameter; C_D0 parameter; rho parameter; c_bar parameter; Rw parameter; r22 parameter; r11 parameter; r00 parameter; z22 parameter; z11 parameter; z00 parameter; zrd parameter
function [F_N,M_rd,d_cp]= fcn(le0, alpha, rot_dot, A_L, A_D, C_D0, rho, c_bar, Rw, r22, r11, r00, z22, z11, z00, zrd)
a2=le0(3)^2+le0(4)^2;
a1=-2*(le0(1)*le0(3)+le0(2)*le0(4));
a0=le0(1)^2+le0(2)^2;
C_L=A_L*sin(2*alpha);
C_D=C_D0+A_D*(1-cos(2*alpha));
C_N=C_L*cos(alpha)+C_D*sin(alpha);
C_A=C_L*sin(alpha)-C_D*cos(alpha);
F_N = -0.5*rho*C_N*c_bar*(a2*Rw^3*r22+a1*Rw^2*r11+a0*Rw*r00);
d_cp_=0.82/pi*(mod(abs(alpha),pi))+0.05;
M_ae=0.5*rho*C_N*c_bar^2*d_cp_*(a2*Rw^3*z22+a1*Rw^2*z11+a0*Rw*z00);
if F_N==0
    d_cp=-0.51*c_bar;
else
    d_cp=M_ae/F_N;
end
M_rd=-0.125*rho*5*rot_dot*abs(rot_dot)*Rw*c_bar^4*zrd;

== matlab function fwv_fulatti/Ref/p,pdot,pddot ==
  data: t input; p output; heading output; v output; a output
function [p,heading , v,a] = fcn(t)
amp=1;
omega=pi/3;
hgt=1;
p=[1 1 1];
if t>0.225
    t=t;
end
heading = 0;
v=[0 0 0];
a=[0 0 0];
% p(1)=amp*sin(omega*t+pi/2)-amp;
% p(2)=amp*sin(omega*t);
% p(3)=hgt;
% v(1)=amp*omega*sin(omega*t+pi);
% v(2)=amp*omega*sin(omega*t+pi/2);
% v(3)=0;
% a(1)=amp*omega*omega*sin(omega*t+3*pi/2);
% a(2)=amp*omega*omega*sin(omega*t+pi);
% a(3)=0;

== matlab function fwv_fulatti/Controller/MATLAB Function ==
  data: Rd output size=[3 3]; mu input; k_hat input; amp output; heading input
function [Rd, amp]= fcn(mu, k_hat,heading)
% k_hat=0.05;
amp=k_hat*(mu(3)+9.806);
if amp > 1
    amp = 1;
end
if amp < 0
    amp = 0;
end
Rz=[cos(heading) -sin(heading) 0;
        sin(heading) cos(heading) 0;
        0 0 1];
% mu=Rz*mu;
mu(3)=9.806;
std_mu=mu./norm(mu);

if norm(std_mu-[0;0;1])<1e-2
    Rd=Rz;
else
    w=cross([0;0;1],std_mu);
    w=w./norm(w);
    theta=acos(dot([0;0;1],std_mu));
    Rd=axang2rotm([w',theta]);
    Rd=Rz * Rd;
end

== matlab function fwv_fulatti/Body/TAIL/get F ==
  data: w input; F output
function F = fcn(w)
l_til=0.01;
A_til=3e-4;
F=-0.5*sign(w)*(0.25*l_til*w)^2*A_til;

== matlab function fwv_fulatti/Controller/period averaging/MATLAB Function ==
  data: R_raw input; R_mean output
function R_mean = fcn(R_raw)
[U,~,V]=svd(R_raw);
R_mean=U*V';

== matlab function fwv_fulatti/Controller/adaptive mapping estimator/update k_hat ==
  data: mu input; k_hat input; k_hat_dot output
function k_hat_dot = fcn(mu,k_hat)
k_hat_dot = 0.005*sign(mu(3))*abs(mu(3))^(1/3);

== matlab function fwv_fulatti/Body/Acuator/ left flap ==
  data: t input; y output; amp input; sig input; freq input; bias input
function y = flap(t,amp,sig,freq,bias)
sig=1-sig;
tn = mod(freq*t,1);
if tn<sig
    y = amp*(cos(2*pi*tn/(2*sig)))+bias;
else
    y = amp*(cos(2*pi*(1-tn)/(2-2*sig)))+bias;
end
if abs(y)>pi/2
    y = sign(y)*pi/2;
end

== matlab function fwv_fulatti/Body/Acuator/ right flap ==
  data: t input; y output; amp input; sig input; freq input; bias input
function y = flap(t,amp,sig,freq,bias)
% sig=1-sig;
tn = mod(freq*t,1);
if tn<sig
    y = amp*(cos(2*pi*tn/(2*sig)))+bias;
else
    y = amp*(cos(2*pi*(1-tn)/(2-2*sig)))+bias;
end
if abs(y)>pi/2
    y = sign(y)*pi/2;
end

== matlab function fwv_fulatti/Controller/slide mode2 ==
  data: u input; y output
function y = fcn(u)

y = sign(u)*abs(u)^(7/9);

== matlab function fwv_fulatti/Body/LEFT WING/AoA ==
  data: le0 input; alpha output; rot input; Rw parameter; r33 parameter; r22 parameter
function alpha = fcn(le0, rot, Rw, r33, r22)
rcp = Rw*r33/r22;
vi = le0(1)+le0(3)*rcp;
vo = le0(2)+le0(4)*rcp;
dir_v = atan2(vo,vi);
if vi~=0
    alpha = -rot + sign(vi)*pi/2 - atan(vo/vi);
else
    alpha = 0;
end
